simulink model "spring_network_AE"  (R2021b)
settings: Solver=FixedStepAuto  StartTime=0.0  StopTime=1e-3  FixedStep=1e-2  RelTol=1e-3
values from neighbouring files (symbols this model uses):
  dq0 = zeros(size(q0))    [simulate_reduced.m]
  q0 = py_encode(xm_mat)    [simulate_reduced.m]
undefined symbols (not defined in the file or in its folder): dynamics_ae
settings Model: Creator=lepri  LastModifiedBy=lepri

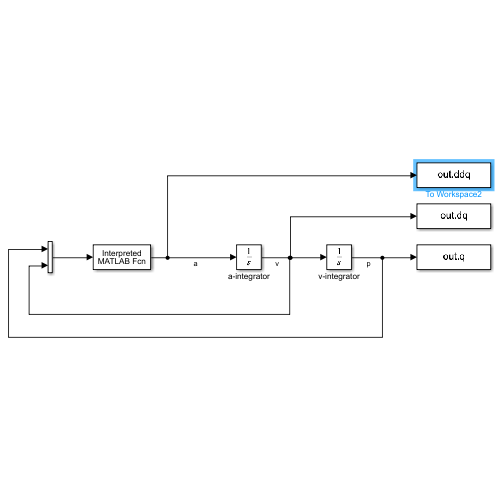
[thumbnail: Simulink's stored preview of the top-level diagram]
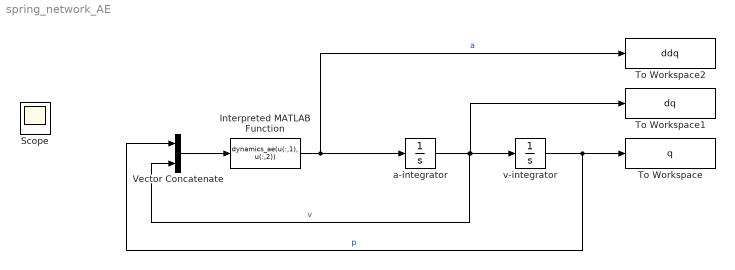
== system spring_network_AE ==
  Interpreted MATLAB Function : MATLABFcn  MATLABFcn=dynamics_ae(u(:,1), u(:,2))
  To Workspace : ToWorkspace  VariableName=q  SampleTime=-1
  To Workspace1 : ToWorkspace  VariableName=dq  SampleTime=-1
  To Workspace2 : ToWorkspace  VariableName=ddq  SampleTime=-1
  Vector Concatenate : Concatenate  Mode=Multidimensional array  ConcatenateDimension=2
  a-integrator : Integrator  InitialCondition=dq0  ContinuousStateAttributes='velocity'
  v-integrator : Integrator  InitialCondition=q0  ContinuousStateAttributes='position'
  Scope : Scope
  wires:
  a-integrator/1 -> To Workspace1/1, v-integrator/1, Vector Concatenate/2  "v"
  v-integrator/1 -> Vector Concatenate/1, To Workspace/1  "p"
  Interpreted MATLAB Function/1 -> To Workspace2/1, a-integrator/1  "a"
  Vector Concatenate/1 -> Interpreted MATLAB Function/1
